simulink model "test_libMdl_Imm"  (R2019b)
settings: Solver=FixedStepDiscrete  StartTime=0  StopTime=50  RelTol=1e-3
PreLoadFcn:
  | init_test_libMdl_Imm
InitFcn:
  | init_test_libMdl_Imm
values from neighbouring files (symbols this model uses):
  Q = cat(3,Q1,Q2)    [init_test_libMdl_Imm.m]
  R = sigma_w^2    (= 1)    [init_test_libMdl_Imm.m]
  sigma_w = 1    [init_test_libMdl_Imm.m]
  T = 0.5    [init_test_libMdl_Imm.m]
  x_02 = [0;10]    [init_test_libMdl_Imm.m]
undefined symbols (not defined in the file or in its folder): mv_seed
libraries: libMdl_Imm x1, dspsrcs4 x1
settings Model: PauseTimes=4.5  Creator=hwinter  LastModifiedBy=Hanno
settings DataIOCC: SaveOutput=off  SignalLogging=off  DSMLogging=off  SaveTime=off  ReturnWorkspaceOutputs=off
settings DebuggingCC: ReadBeforeWriteMsg=DisableAll  WriteAfterWriteMsg=DisableAll  WriteAfterReadMsg=DisableAll  MultiTaskDSMMsg=none  ArithmeticOperatorsInVariantConditions=warning
settings HardwareCC: ProdBitPerLong=64  ProdHWDeviceType=Intel->x86-64 (Linux 64)  TargetBitPerPointer=64  TargetBitPerSizeT=64  TargetBitPerPtrDiffT=64  TargetLongLongMode=on  TargetIntDivRoundTo=Zero  TargetEndianess=LittleEndian  TargetWordSize=64  TargetHWDeviceType=MATLAB Host  ProdEqTarget=off
settings SFSimCC: SFSimEcho=off  SimUseLocalCustomCode=off  CustomCodeUndefinedFunction=UseInterfaceOnly
settings RTWCC: Description=Rapid Simulation Target  SystemTargetFile=rsim.tlc  TemplateMakefile=rsim_default_tmf  RTWUseLocalCustomCode=off
settings CodeAppCC: StateflowObjectComments=on
settings RSimTargetCC: TargetLangStandard=C99 (ISO)  GeneratePreprocessorConditionals=Use local settings  PreserveStateflowLocalDataDimensions=off

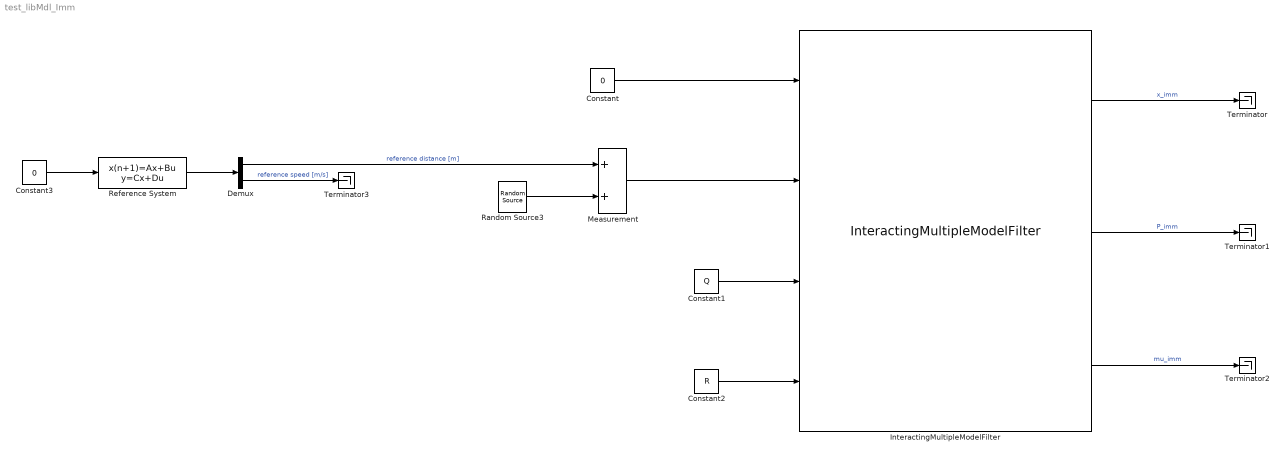
== system test_libMdl_Imm ==
  Constant : Constant  Value=0
  Constant1 : Constant  Value=Q
  Constant2 : Constant  Value=R
  Constant3 : Constant  Value=0
  Demux : Demux  Outputs=2
  InteractingMultipleModelFilter : libMdl_Imm/InteractingMultipleModelFilter  mv_sample_time=T  mv_x_0=x_0  mv_P_0=P_0  mv_pi=Pi  mv_mu_0=mu_0  mv_state_transition_functions=state_transition_fcns  mv_measurement_functions=measurement_fcns
  Measurement : Sum
  Random Source3 : dspsrcs4/Random Source  SrcType=Gaussian  NormMethod=Ziggurat  CltLength=12  MinVal=0  MaxVal=1  MeanVal=0  VarVal=sigma_w^2  RepMode=Not repeatable  rawSeed=mv_seed+1  IsInherit=on  SampMode=Discrete  SampTime=1  SampFrame=1  DataType=Double  OutComplex=Real  OutputFrames=off
  Reference System : DiscreteStateSpace  A=[1 T;0 1]  B=[0;0]  C=[1 0;0 1]  D=[0;0]  InitialCondition=x_02  SampleTime=T
  Terminator{,1..3} (4 alike) : Terminator
  wires:
  InteractingMultipleModelFilter/1 -> Terminator/1  "x_imm"
  InteractingMultipleModelFilter/2 -> Terminator1/1  "P_imm"
  InteractingMultipleModelFilter/3 -> Terminator2/1  "mu_imm"
  Demux/2 -> Terminator3/1  "reference speed [m/s]"
  Measurement/1 -> InteractingMultipleModelFilter/2
  Demux/1 -> Measurement/1  "reference distance [m]"
  Constant1/1 -> InteractingMultipleModelFilter/3
  Constant2/1 -> InteractingMultipleModelFilter/4
  Constant3/1 -> Reference System/1
  Random Source3/1 -> Measurement/2
  Constant/1 -> InteractingMultipleModelFilter/1
  Reference System/1 -> Demux/1
